simulink model "shem2"  (R2023a)
settings: Solver=VariableStepAuto  StartTime=0.0  StopTime=10.0  RelTol=1e-3
settings Model: Creator=fynjy  LastModifiedBy=fynjy

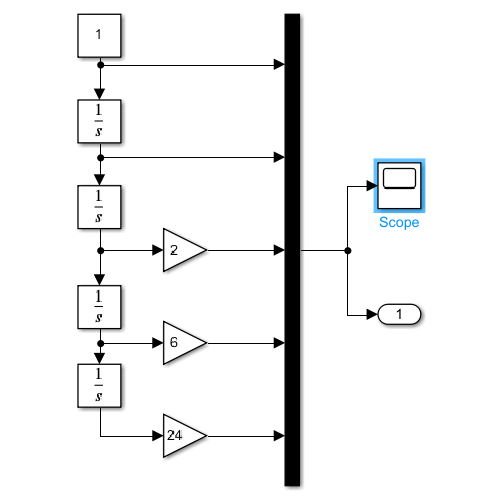
[thumbnail: Simulink's stored preview of the top-level diagram]
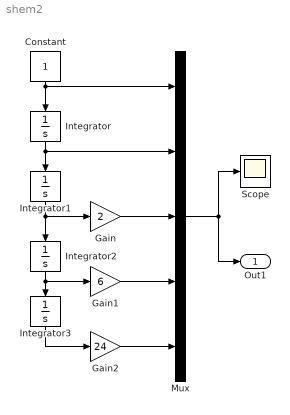
== system shem2 ==
  Constant : Constant
  Gain : Gain  Gain=2
  Gain1 : Gain  Gain=6
  Gain2 : Gain  Gain=24
  Integrator{,1..3} (4 alike) : Integrator
  Mux : Mux  Inputs=5
  Scope : Scope
  Out1 : Outport
  wires:
  Constant/1 -> Mux/1, Integrator/1
  Integrator/1 -> Integrator1/1, Mux/2
  Mux/1 -> Out1/1, Scope/1
  Integrator1/1 -> Gain/1, Integrator2/1
  Integrator2/1 -> Gain1/1, Integrator3/1
  Integrator3/1 -> Gain2/1
  Gain2/1 -> Mux/5
  Gain1/1 -> Mux/4
  Gain/1 -> Mux/3
